simulink model "Park_Clark"  (R2022b)
settings: Solver=VariableStepAuto  StartTime=0.0  StopTime=10.0  RelTol=1e-3
settings Model: Creator=emate  LastModifiedBy=emate

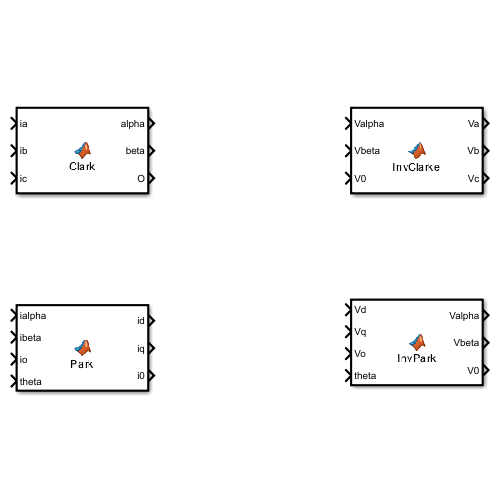
[thumbnail: Simulink's stored preview of the top-level diagram]
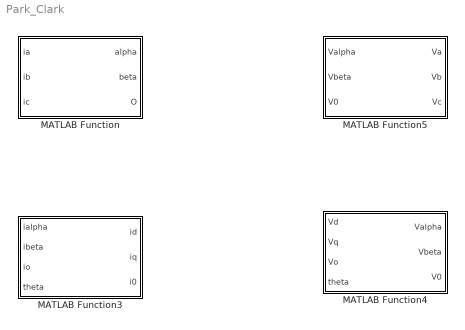
== system Park_Clark ==
  MATLAB Function : MATLAB Function  TreatAsAtomicUnit=on
  MATLAB Function3 : MATLAB Function  TreatAsAtomicUnit=on
  MATLAB Function4 : MATLAB Function  TreatAsAtomicUnit=on
  MATLAB Function5 : MATLAB Function  TreatAsAtomicUnit=on

== matlab function Park_Clark/MATLAB Function ==
  data: ia input; alpha output; ib input; beta output; ic input; O output
function [alpha,beta,O] = Clark(ia,ib,ic)

alpha =  2/3 * (ia - 0.5*ib - 0.5*ic);

beta  =  2/3 * (((sqrt(3)*ib)/2) + (-(sqrt(3)*ic)/2));

O     =  2/3 * (0.5*ia + 0.5*ib + 0.5*ic);

== matlab function Park_Clark/MATLAB Function3 ==
  data: ialpha input; id output; ibeta input; io input; iq output; theta input; i0 output
function [id,iq,i0] = Park(ialpha,ibeta,io,theta)

s=sin(theta);
c=cos(theta);

id = c * ialpha + s * ibeta;

iq = -s * ialpha + c * ibeta;

i0 = io;

== matlab function Park_Clark/MATLAB Function4 ==
  data: Vd input; Valpha output; Vq input; Vo input; Vbeta output; theta input; V0 output
function [Valpha,Vbeta,V0] = InvPark(Vd,Vq,Vo,theta)

c=cos(theta);
s=sin(theta);

Valpha = Vd*c - Vq*s;

Vbeta = Vq*c + Vd*s;

V0 = Vo;

== matlab function Park_Clark/MATLAB Function5 ==
  data: Valpha input; Va output; Vbeta input; Vb output; Vc output; V0 input
function [Va,Vb,Vc] = InvClarke(Valpha,Vbeta,V0)

Va = Valpha + V0;

Vb = -0.5*Valpha + (sqrt(3)/2)*Vbeta + V0;

Vc = -0.5*Valpha - (sqrt(3)/2)*Vbeta + V0;
